simulink model "Bicycle_IO"  (R2024b)
settings: Solver=VariableStepAuto  StartTime=0.0  StopTime=T  RelTol=1e-3
undefined symbols (not defined in the file): L, theta_i, x_i, y_i
libraries: robotmobilelib x1, sim3dlib x1, sim3dautolib x1
settings Model: Creator=loren  LastModifiedBy=loren

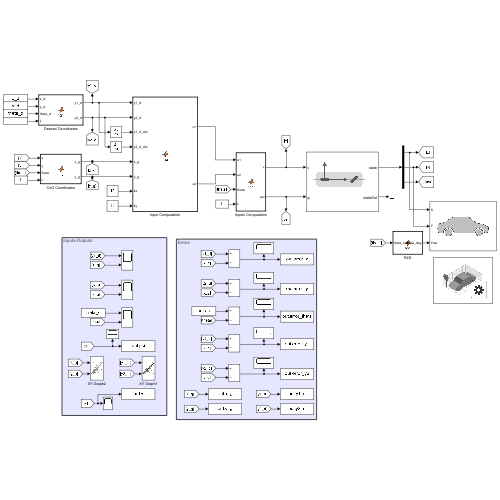
[thumbnail: Simulink's stored preview of the top-level diagram]
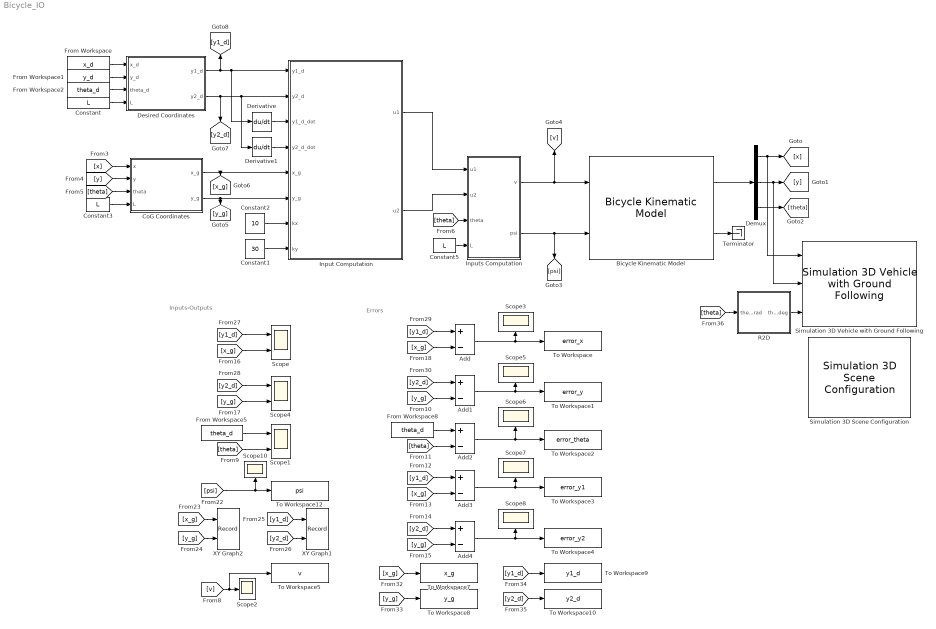
== system Bicycle_IO ==
  note: Inputs-Outputs
  note: Errors
  Add{,1..4} (5 alike) : Sum  Inputs=+-
  Bicycle Kinematic Model : robotmobilelib/Bicycle Kinematic Model  VehicleInputs=Vehicle Speed & Steering Angle  WheelBase=L  VehicleSpeedRange=[-10, 10]  MaxSteeringAngle=pi/3  InitialState=q_i  SimulateUsing=Interpreted execution
  CoG Coordinates : MATLAB Function  TreatAsAtomicUnit=on
  Constant : Constant  Value=L
  Constant1 : Constant  Value=30
  Constant2 : Constant  Value=10
  Constant3 : Constant  Value=L
  Constant5 : Constant  Value=L
  Demux : Demux  Outputs=3
  Derivative : Derivative
  Derivative1 : Derivative
  Desired Coordinates : MATLAB Function  TreatAsAtomicUnit=on
  From Workspace : FromWorkspace  VariableName=x_d
  From Workspace1 : FromWorkspace  VariableName=y_d
  From Workspace2 : FromWorkspace  VariableName=theta_d
  From Workspace5 : FromWorkspace  VariableName=theta_d
  From Workspace8 : FromWorkspace  VariableName=theta_d
  Input Computation : MATLAB Function  TreatAsAtomicUnit=on
  Inputs Computation : MATLAB Function  TreatAsAtomicUnit=on
  R2D : MATLAB Function  TreatAsAtomicUnit=on
  Scope : Scope  NumInputPorts=2
  Scope1 : Scope  NumInputPorts=2
  Scope{2..3,5..8,10} (7 alike) : Scope
  Scope4 : Scope  NumInputPorts=2
  Simulation 3D Scene Configuration : sim3dlib/Simulation 3D Scene Configuration  Priority=0  ProjectFormat=Default Scenes  SceneDesc=Open surface  ProjectName=C:\Program Files\MATLAB\R2024b\toolbox\shared\sim3d_projects\automotive_project_windows\UE\WindowsNoEditor\VehicleSimulation.exe  ScenePath=/Game/Maps/HwStrght  EnableOpenDRIVE=off  vehTagList={'Custom';'Scene Origin';'SimulinkVehicle1'}  vehTag=SimulinkVehicle1  FreeCameraInitialTranslation=[0, 0, 0]  FreeCameraDefaultInitialTranslation=[-6, 0, 2]  FreeCameraInitialRotation=[0, 0, 0]  FreeCameraDefaultInitialRotation=[0, -15, 0]  OpVisEn=off  Ts=.02  EnableWindow=on  EnableRemoteAccess=off  EnableWeather=off  SunAzimuth=90  SunAltitude=40.0  EnableGeospatialSun=off  Latitude=0  Longitude=0  Date=2023-01-01  Time=10:30:00  GeoTimeZone=-5.0  SunDaylightSaving=off  wind=1  clouds=10  EnableVolumetricClouds=off  CloudCoverage=0  CloudAltitude=6  fog=0  rain=0  RaindropsEffect=off  SnowDensity=0  EnableGeospatial=off  UseTrueOrigin=off  OriginHeight=200  OriginLatitude=40.744652  OriginLongitude=-73.988864  MapStyle=Aerial  AdditionalAssetIDs=[]  UseAdvancedSunSky=off  SolarTime=11  TimeZone=-5  Day=21  Month=9  Year=2022  UseDaylightSavingTime=on  DSTStartDay=10  DSTStartMonth=3  DSTEndDay=3  DSTEndMonth=11  DSTSwitchHour=2  sensorTag=MainCamera1  sensorId=1  sensorName=MainCamera1  mountLoc=Origin  offsetFlag=off  tmountOffset=[0, 0, 0]  rmountOffset=[0, 0, 0]  HorizontalResolution=1280  VerticalResolution=720  HorizontalFOV=60  mountPoint=[0 0 0]  mountOrientation=[0 0 0]  aMode=2  ID=1  GeoTrigger=Inactive
      settings: LibrarySourceBlock=vehdynlibsim3dcore/Simulation 3D Scene Configuration
  Simulation 3D Vehicle with Ground Following : sim3dautolib/Simulation 3D Vehicle with Ground Following  Priority=-1  PassVehMesh=Sedan  MeshPath=/MathWorksAutomotiveContent/Vehicles/Muscle/Meshes/SK_MuscleCar.SK_MuscleCar  TrackWidth=1.9  WheelBase=3  WheelRadius=0.35  VehColor=Black  InitialPos=[x_i, y_i, 0]  InitialRot=[0, 0, theta_i*180/pi]  ActorName=SimulinkVehicle1  SampleTime=0.01  ActorType=SimulinkVehicle  ID=1  aMode=3  ActorTag=SimulinkVehicle1  CoordinateScheme=ISO  VehLightsControl=off  HeadlightColor=[ 1, 1, 1 ]  HighBeamIntensity=100000  LowBeamIntensity=60000  HighBeamConeAngle=70  LowBeamConeAngle=70  LeftHeadlightOrientation=[ 0, 0 ]  RightHeadlightOrientation=[ 0, 0 ]  BrakelightIntensity=500  ReverselightIntensity=500  SignallightIntensity=500  SignallightPeriod=1  SignalPulseWidth=50  TransformOutportEnabled=off
      settings: LibrarySourceBlock=drivingsim3d/Simulation 3D Vehicle with Ground Following
  Terminator : Terminator
  To Workspace : ToWorkspace  VariableName=error_x  SaveFormat=Timeseries  SampleTime=-1
  To Workspace1 : ToWorkspace  VariableName=error_y  SaveFormat=Timeseries  SampleTime=-1
  To Workspace10 : ToWorkspace  VariableName=y2_d  SaveFormat=Timeseries  SampleTime=-1
  To Workspace12 : ToWorkspace  VariableName=psi  SaveFormat=Timeseries  SampleTime=-1
  To Workspace2 : ToWorkspace  VariableName=error_theta  SaveFormat=Timeseries  SampleTime=-1
  To Workspace3 : ToWorkspace  VariableName=error_y1  SaveFormat=Timeseries  SampleTime=-1
  To Workspace4 : ToWorkspace  VariableName=error_y2  SaveFormat=Timeseries  SampleTime=-1
  To Workspace5 : ToWorkspace  VariableName=v  SaveFormat=Timeseries  SampleTime=-1
  To Workspace7 : ToWorkspace  VariableName=x_g  SaveFormat=Timeseries  SampleTime=-1
  To Workspace8 : ToWorkspace  VariableName=y_g  SaveFormat=Timeseries  SampleTime=-1
  To Workspace9 : ToWorkspace  VariableName=y1_d  SaveFormat=Timeseries  SampleTime=-1
  XY Graph1 : Record  FileSettingsInternal="{\"entries\":[{\"content\":{\"excelSettings\":{\"content\":{},\"type\":\"Streamout.ExcelSettings\"}},\"type\":\"Streamout.FileSettingStorage\",\"uuid\":\"\"}],\"packageUris\":[\"http:\\/\\/schema.mathworks.com\\/mf0\\/streamout_blocks\\/R2020a\"],\"version\":\"1.0\"}"  Layout=[1 1]  SignalsInternal="{\"entries\":[{\"content\":{\"signals\":[{\"content\":{\"blockPath\":[],\"dimensions\":[1],\"domain\":\"\",\"lineColor\":\"#a2142f\",\"plots\":[ 1 ],\"port\":1,\"sid\":[\"\"],\"signalID\":1,\"signalName\":\"From25\"},\"type\":\"RecordBlkView.Signal\",\"uuid\":\"\"},{\"content\":{\"blockPath\":[],\"dimensions\":[1],\"domain\":\"\",\"lineColor\":\"#139fff\",\"plots\":[ 1 ],\"port\":2,\"sid\":[\"\"],\"signalID\":2,\"signalName\":\"From26\"},\"type\":\"RecordBlkView.Signal\",\"uuid\":\"\"}]},\"type\":\"RecordBlkView.InputSignals\",\"uuid\":\"\"}],\"packageUris\":[\"http:\\/\\/schema.mathworks.com\\/mf0\\/streamout_blocks\\/R2020a\"],\"version\":\"1.0\"}"  VisualizationBindings="{\"xyplotplugin\":{\"info\":[{\"series\":[{\"bindingParametersList\":[{\"parameter\":\"X-Axis\",\"signalID\":1,\"signalName\":\"From25\"},{\"parameter\":\"Y-Axis\",\"signalID\":2,\"signalName\":\"From26\"}],\"seriesID\":0}],\"subplotID\":1}]}}"  CompatibilityTag=XY
  XY Graph2 : Record  FileSettingsInternal="{\"entries\":[{\"content\":{\"excelSettings\":{\"content\":{},\"type\":\"Streamout.ExcelSettings\"}},\"type\":\"Streamout.FileSettingStorage\",\"uuid\":\"\"}],\"packageUris\":[\"http:\\/\\/schema.mathworks.com\\/mf0\\/streamout_blocks\\/R2020a\"],\"version\":\"1.0\"}"  Layout=[1 1]  SignalsInternal="{\"entries\":[{\"content\":{\"signals\":[{\"content\":{\"blockPath\":[],\"dimensions\":[1],\"domain\":\"\",\"lineColor\":\"#fe330a\",\"lineWidth\":2,\"port\":1,\"sid\":[\"\"],\"signalID\":1,\"signalName\":\"From23\"},\"type\":\"RecordBlkView.Signal\",\"uuid\":\"\"},{\"content\":{\"blockPath\":[],\"dimensions\":[1],\"domain\":\"\",\"lineColor\":\"#22b573\",\"lineWidth\":2,\"port\":2,\"sid\":[\"\"],\"signalID\":2,\"signalName\":\"From24\"},\"type\":\"RecordBlkView.Signal\",\"uuid\":\"\"}]},\"type\":\"RecordBlkView.InputSignals\",\"uuid\":\"\"}],\"packageUris\":[\"http:\\/\\/schema.mathworks.com\\/mf0\\/streamout_blocks\\/R2020a\"],\"version\":\"1.0\"}"  VisualizationBindings="{\"xyplotplugin\":{\"info\":[{\"series\":[],\"subplotID\":1}]}}"  CompatibilityTag=XY
  wires:
  [x] -> CoG Coordinates/1(x)
  [x_g] -> Add/2
  CoG Coordinates/2(y_g) -> Input Computation/6(y_g), [y_g]
  [y2_d] -> Add1/1
  [x_g] -> Add3/2
  Bicycle Kinematic Model/2 -> Terminator/1
  Constant2/1 -> Input Computation/7(kx)
  Add/1 -> To Workspace/1, Scope3/1
  [y_g] -> Add4/2
  [theta] -> CoG Coordinates/3(theta)
  [v] -> To Workspace5/1, Scope2/1
  From Workspace2/1 -> Desired Coordinates/3(theta_d)
  Input Computation/1(u1) -> Inputs Computation/1(u1)
  Add1/1 -> To Workspace1/1, Scope5/1
  [y1_d] -> Scope/1
  Desired Coordinates/1(y1_d) -> [y1_d], Derivative/1, Input Computation/1(y1_d)
  CoG Coordinates/1(x_g) -> [x_g], Input Computation/5(x_g)
  Bicycle Kinematic Model/1 -> Demux/1
  From Workspace8/1 -> Add2/1
  [y2_d] -> Add4/1
  [theta] -> Scope1/2
  Input Computation/2(u2) -> Inputs Computation/2(u2)
  [y2_d] -> Scope4/1
  [y1_d] -> Add3/1
  [y1_d] -> Add/1
  [theta] -> Add2/2
  Add2/1 -> To Workspace2/1, Scope6/1
  Demux/2 -> Simulation 3D Vehicle with Ground Following/2, [y]
  Constant1/1 -> Input Computation/8(ky)
  Demux/3 -> [theta]
  Add3/1 -> To Workspace3/1, Scope7/1
  [x_g] -> Scope/2
  Demux/1 -> [x], Simulation 3D Vehicle with Ground Following/1
  [theta] -> Inputs Computation/3(theta)
  [y] -> CoG Coordinates/2(y)
  [y_g] -> Add1/2
  [y_g] -> Scope4/2
  Desired Coordinates/2(y2_d) -> [y2_d], Derivative1/1, Input Computation/2(y2_d)
  Add4/1 -> To Workspace4/1, Scope8/1
  From Workspace5/1 -> Scope1/1
  Derivative/1 -> Input Computation/3(y1_d_dot)
  Derivative1/1 -> Input Computation/4(y2_d_dot)
  Constant/1 -> Desired Coordinates/4(L)
  Constant3/1 -> CoG Coordinates/4(L)
  Constant5/1 -> Inputs Computation/4(L)
  [psi] -> To Workspace12/1, Scope10/1
  [x_g] -> XY Graph2/1
  [y_g] -> XY Graph2/2
  [y2_d] -> XY Graph1/2
  [y1_d] -> XY Graph1/1
  Inputs Computation/1(v) -> [v], Bicycle Kinematic Model/1
  Inputs Computation/2(psi) -> Bicycle Kinematic Model/2, [psi]
  [x_g] -> To Workspace7/1
  [y_g] -> To Workspace8/1
  [y1_d] -> To Workspace9/1
  [y2_d] -> To Workspace10/1
  R2D/1(theta_deg) -> Simulation 3D Vehicle with Ground Following/3
  [theta] -> R2D/1(theta_rad)
  From Workspace/1 -> Desired Coordinates/1(x_d)
  From Workspace1/1 -> Desired Coordinates/2(y_d)

== matlab function Bicycle_IO/R2D ==
  data: theta_rad input; theta_deg output
function theta_deg = fcn(theta_rad)

theta_deg = theta_rad*180/pi;

== matlab function Bicycle_IO/CoG Coordinates ==
  data: x input; x_g output; y input; theta input; y_g output; L input
function [x_g, y_g] = fnc(x, y, theta, L)

b = L/2;

x_g = x + b * cos(theta);
y_g = y + b * sin(theta);

== matlab function Bicycle_IO/Input Computation ==
  data: y1_d input; u1 output; y2_d input; y1_d_dot input; y2_d_dot input; x_g input; y_g input; kx input; ky input; u2 output
function [u1, u2] = fnc(y1_d, y2_d, y1_d_dot, y2_d_dot, x_g, y_g, kx, ky)

u1 = y1_d_dot + kx*(y1_d - x_g); 
u2 = y2_d_dot + ky*(y2_d - y_g);

== matlab function Bicycle_IO/Desired Coordinates ==
  data: x_d input; y1_d output; y_d input; theta_d input; y2_d output; L input
function [y1_d, y2_d] = fcn(x_d, y_d, theta_d, L)

b = L/2;

y1_d = x_d + b * cos(theta_d);
y2_d = y_d + b * sin(theta_d);

== matlab function Bicycle_IO/Inputs Computation ==
  data: u1 input; v output; u2 input; theta input; psi output; L input
function [v, psi] = fcn(u1, u2, theta, L)

b = L/2;

A = [cos(theta),   -b*sin(theta);
     sin(theta),    b*cos(theta)]; % It's invertible since L > 0 always

A_inverse = inv(A);

v = A_inverse(1,:)*[u1; u2];
theta_dot = A_inverse(2,:)*[u1; u2];

    if abs(v) > 1e-6  % Avoid singularity
        psi = atan((theta_dot * L) / v);
    else
        psi = 0;
    end

    % Maximum feasible limit for psi
 psi_max = 60 * pi/180;  % ±60 degrees
 psi = max(-psi_max, min(psi_max, psi));
